simulink model "Spektren_Digitale_Modulation"  (Simulink 8.6)
settings: Solver=FixedStepDiscrete  StartTime=0  StopTime=inf  RelTol=1e-3
undefined symbols (not defined in the file or in its folder): gcbh, magnitude, rcfiltgaincompat
libraries: commfilt2 x6, commrandsrc2 x6, commdigbbndam3 x4, dspstat3 x3, commdigbbndpm3 x2, dspsigops x1, simulink x1
settings Model: Creator=schwall  LastModifiedBy=wunsch
settings DataIOCC: SaveOutput=off  SignalLogging=off  SaveTime=off
settings DebuggingCC: FcnCallInpInsideContextMsg=UseLocalSettings

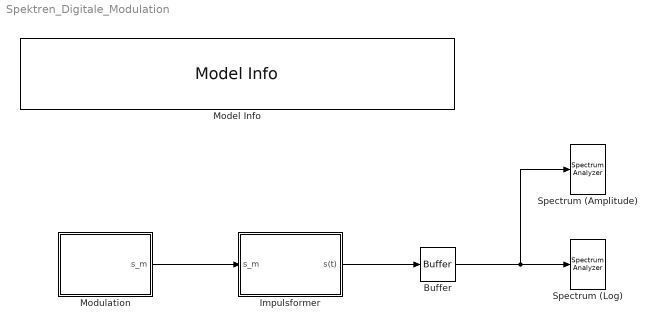
== system Spektren_Digitale_Modulation ==
  Buffer : Buffer  N=1024
  Impulsformer : Subsystem  mask(Impulsformer){rolloff_set=0.4}
      mask prompts: rolloff_set "Root-Raised Cosinus Filter, Roll-Off Faktor:"
      mask help: Impulsformer auswaehlen. Zweiter Vektor ist Rechteckimpulsform.
      mask TypeOptions rolloff_set: 0 | 0.2 | 0.4 | 0.6 | 0.8 | 1
  Model Info : simulink/Model-Wide Utilities/Model Info  BlockCM=None  Frame=on  DisplayStringWithTags=|  HorizontalTextAlignment=Left  LeftAlignmentValue=0.02  SourceBlockDiagram=Spektren_Digitale_Modulation  TagMaxNumber=20
      | Demo Spektren Digitale Modulation
      | Vorlesung Nachrichtentechnik II
      | Institut fuer Nachrichtentechnik (CEL)
  Modulation : Subsystem  mask(Modulation){mod_set=QPSK, mod_prob=0.5, fs=1/100, P=1}
      mask prompts: mod_set "Modulationsverfahren:"; mod_prob "Wahrscheinlichkeit fuer binaere Null:"; fs "Symboldauer [s]:"; P "Leistung, bezogen auf 1 Ohm [Watt]"
      mask help: Modulationsverfahren auswaehlen.
      mask TypeOptions mod_set: 2-ASK | QPSK | 16-PSK | 4-QAM | 16-QAM | 256-QAM
  Spectrum (Amplitude) : SpectrumAnalyzer
  Spectrum (Log) : SpectrumAnalyzer
  wires:
  Modulation/1(s_m) -> Impulsformer/1(s_m)
  Buffer/1 -> Spectrum (Log)/1, Spectrum (Amplitude)/1
  Impulsformer/1(s(t)) -> Buffer/1

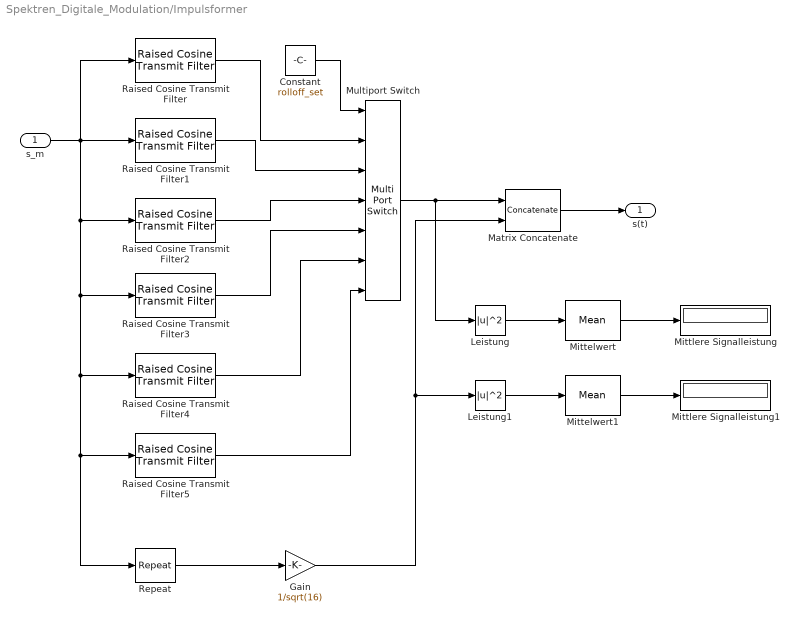
== system Spektren_Digitale_Modulation/Impulsformer ==
  s_m : Inport
  Constant : Constant  Value=rolloff_set
  Gain : Gain  Gain=1/sqrt(16)
  Leistung : Math  Operator=magnitude^2  SaturateOnIntegerOverflow=on
  Leistung1 : Math  Operator=magnitude^2  SaturateOnIntegerOverflow=on
  Matrix Concatenate : Concatenate  Mode=Multidimensional array  ConcatenateDimension=2
  Mittelwert : dspstat3/Mean  run=on  reset_popup=None  InputProcessing=Inherited (this choice will be removed - see release notes)  directionMode=Each column  dimension=1  roiEnable=off  roiType=Rectangles  roiPortion=Entire ROI  roiOutput=Individual statistics for each ROI  roiFlag=off  outputDataTypeStr=Inherit: Same as accumulator  outputLastDataTypeStr=Inherit: Same as accumulator  outputMin=[]  outputMax=[]  roundingMode=Floor  overflowMode=off
  Mittelwert1 : dspstat3/Mean  run=on  reset_popup=None  InputProcessing=Inherited (this choice will be removed - see release notes)  directionMode=Each column  dimension=1  roiEnable=off  roiType=Rectangles  roiPortion=Entire ROI  roiOutput=Individual statistics for each ROI  roiFlag=off  outputDataTypeStr=Inherit: Same as accumulator  outputLastDataTypeStr=Inherit: Same as accumulator  outputMin=[]  outputMax=[]  roundingMode=Floor  overflowMode=off
  Mittlere Signalleistung : Display
  Mittlere Signalleistung1 : Display
  Multiport Switch : MultiPortSwitch  Inputs=6
  Raised Cosine Transmit Filter : commfilt2/Raised Cosine Transmit Filter  filtType=Square root  filtSpan=2*(6)  currentFiltSpan=2*(6)  D=6  R=0  sampMode=Mute  saveAsFlag=0  N=16  framing=Maintain input frame rate  InputProcessing=Columns as channels (frame based)  checkGain=Normalized  filterGain=rcfiltgaincompat(gcbh)  checkCoeff=off  variableName=rcTxFilt  launchFVT=off  roundingMode=Floor  overflowMode=off
  Raised Cosine Transmit Filter1 : commfilt2/Raised Cosine Transmit Filter  filtType=Square root  filtSpan=2*(6)  currentFiltSpan=2*(6)  D=6  R=0.2  sampMode=Mute  saveAsFlag=0  N=16  framing=Maintain input frame rate  InputProcessing=Columns as channels (frame based)  checkGain=Normalized  filterGain=rcfiltgaincompat(gcbh)  checkCoeff=off  variableName=rcTxFilt1  launchFVT=off  roundingMode=Floor  overflowMode=off
  Raised Cosine Transmit Filter2 : commfilt2/Raised Cosine Transmit Filter  filtType=Square root  filtSpan=2*(6)  currentFiltSpan=2*(6)  D=6  R=0.4  sampMode=Mute  saveAsFlag=0  N=16  framing=Maintain input frame rate  InputProcessing=Columns as channels (frame based)  checkGain=Normalized  filterGain=rcfiltgaincompat(gcbh)  checkCoeff=off  variableName=rcTxFilt2  launchFVT=off  roundingMode=Floor  overflowMode=off
  Raised Cosine Transmit Filter3 : commfilt2/Raised Cosine Transmit Filter  filtType=Square root  filtSpan=2*(6)  currentFiltSpan=2*(6)  D=6  R=0.6  sampMode=Mute  saveAsFlag=0  N=16  framing=Maintain input frame rate  InputProcessing=Columns as channels (frame based)  checkGain=Normalized  filterGain=rcfiltgaincompat(gcbh)  checkCoeff=off  variableName=rcTxFilt3  launchFVT=off  roundingMode=Floor  overflowMode=off
  Raised Cosine Transmit Filter4 : commfilt2/Raised Cosine Transmit Filter  filtType=Square root  filtSpan=2*(6)  currentFiltSpan=2*(6)  D=6  R=0.8  sampMode=Mute  saveAsFlag=0  N=16  framing=Maintain input frame rate  InputProcessing=Columns as channels (frame based)  checkGain=Normalized  filterGain=rcfiltgaincompat(gcbh)  checkCoeff=off  variableName=rcTxFilt4  launchFVT=off  roundingMode=Floor  overflowMode=off
  Raised Cosine Transmit Filter5 : commfilt2/Raised Cosine Transmit Filter  filtType=Square root  filtSpan=2*(6)  currentFiltSpan=2*(6)  D=6  R=1  sampMode=Mute  saveAsFlag=0  N=16  framing=Maintain input frame rate  InputProcessing=Columns as channels (frame based)  checkGain=Normalized  filterGain=rcfiltgaincompat(gcbh)  checkCoeff=off  variableName=rcTxFilt5  launchFVT=off  roundingMode=Floor  overflowMode=off
  Repeat : dspsigops/Repeat  N=16  InputProcessing=Inherited (this choice will be removed - see release notes)  RateOptions=Enforce single-rate processing  ic=0  mode=Unused parameter value
  s(t) : Outport
  wires:
  s_m/1 -> Raised Cosine Transmit Filter/1, Raised Cosine Transmit Filter5/1, Repeat/1, Raised Cosine Transmit Filter4/1, Raised Cosine Transmit Filter3/1, Raised Cosine Transmit Filter2/1, Raised Cosine Transmit Filter1/1
  Mittelwert/1 -> Mittlere Signalleistung/1
  Leistung/1 -> Mittelwert/1
  Mittelwert1/1 -> Mittlere Signalleistung1/1
  Leistung1/1 -> Mittelwert1/1
  Multiport Switch/1 -> Matrix Concatenate/1, Leistung/1
  Constant/1 -> Multiport Switch/1
  Raised Cosine Transmit Filter/1 -> Multiport Switch/2
  Raised Cosine Transmit Filter1/1 -> Multiport Switch/3
  Raised Cosine Transmit Filter2/1 -> Multiport Switch/4
  Raised Cosine Transmit Filter3/1 -> Multiport Switch/5
  Raised Cosine Transmit Filter4/1 -> Multiport Switch/6
  Raised Cosine Transmit Filter5/1 -> Multiport Switch/7
  Gain/1 -> Leistung1/1, Matrix Concatenate/2
  Repeat/1 -> Gain/1
  Matrix Concatenate/1 -> s(t)/1

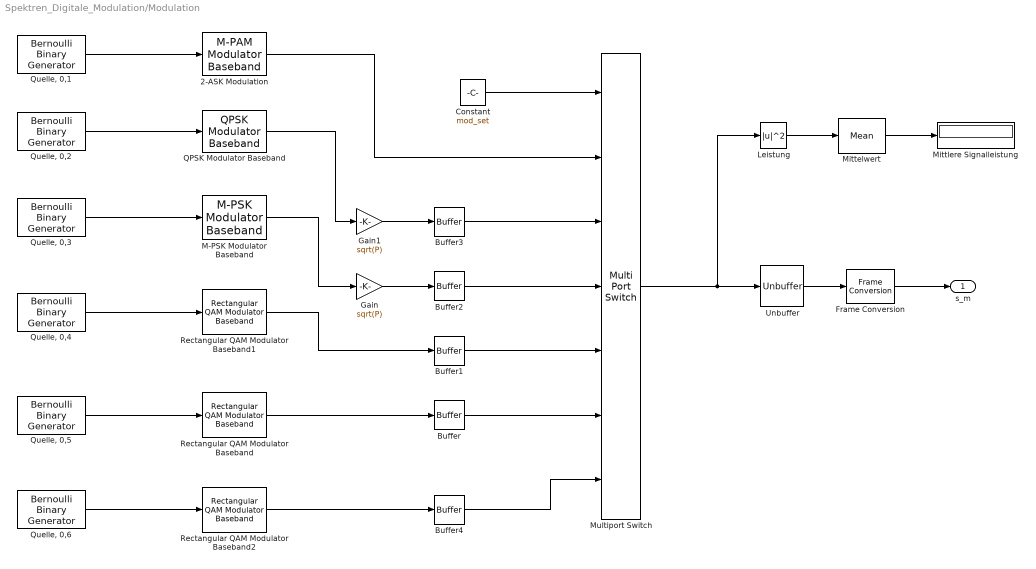
== system Spektren_Digitale_Modulation/Modulation ==
  2-ASK Modulation : commdigbbndam3/M-PAM Modulator Baseband  M=2  InType=Integer  Enc=Binary  PowType=Average Power  MinDist=2  AvgPow=P  PeakPow=1  outDtype=double  outWordLen=16  outUDDataType=sfix(16)  outFracLenMode=Best precision  outFracLen=15
  Buffer{,1..4} (5 alike) : Buffer  N=8
  Constant : Constant  Value=mod_set
  Frame Conversion : FrameConversion  InheritSamplingMode=off
  Gain : Gain  Gain=sqrt(P)
  Gain1 : Gain  Gain=sqrt(P)
  Leistung : Math  Operator=magnitude^2  SaturateOnIntegerOverflow=on
  M-PSK Modulator Baseband : commdigbbndpm3/M-PSK Modulator Baseband  M=16  InType=Bit  Enc=Gray  Mapping=[0:7]  Ph=pi/8  outDtype=double  outWordLen=16  outUDDataType=sfix(16)  outFracLenMode=Best precision  outFracLen=15
  Mittelwert : dspstat3/Mean  run=on  reset_popup=None  InputProcessing=Inherited (this choice will be removed - see release notes)  directionMode=Each column  dimension=1  roiEnable=off  roiType=Rectangles  roiPortion=Entire ROI  roiOutput=Individual statistics for each ROI  roiFlag=off  outputDataTypeStr=Inherit: Same as accumulator  outputLastDataTypeStr=Inherit: Same as accumulator  outputMin=[]  outputMax=[]  roundingMode=Floor  overflowMode=off
  Mittlere Signalleistung : Display
  Multiport Switch : MultiPortSwitch  Inputs=6
  QPSK Modulator Baseband : commdigbbndpm3/QPSK Modulator Baseband  InType=Bit  Enc=Gray  Ph=0  outDtype=double  outWordLen=16  outUDDataType=sfix(16)  outFracLenMode=Best precision  outFracLen=15
  "Quelle, 0,1" : commrandsrc2/Bernoulli Binary Generator  P=mod_prob  seed=61  Ts=fs  frameBased=on  sampPerFrame=8  orient=off  outDataType=double
  "Quelle, 0,2" : commrandsrc2/Bernoulli Binary Generator  P=mod_prob  seed=61  Ts=fs/2  frameBased=on  sampPerFrame=8  orient=off  outDataType=double
  "Quelle, 0,3" : commrandsrc2/Bernoulli Binary Generator  P=mod_prob  seed=61  Ts=fs/4  frameBased=on  sampPerFrame=8  orient=off  outDataType=double
  "Quelle, 0,4" : commrandsrc2/Bernoulli Binary Generator  P=mod_prob  seed=61  Ts=fs/2  frameBased=on  sampPerFrame=8  orient=off  outDataType=double
  "Quelle, 0,5" : commrandsrc2/Bernoulli Binary Generator  P=mod_prob  seed=61  Ts=fs/4  frameBased=on  sampPerFrame=8  orient=off  outDataType=double
  "Quelle, 0,6" : commrandsrc2/Bernoulli Binary Generator  P=mod_prob  seed=61  Ts=fs/8  frameBased=on  sampPerFrame=8  orient=off  outDataType=double
  Rectangular QAM Modulator Baseband : commdigbbndam3/Rectangular QAM Modulator Baseband  M=16  InType=Bit  Enc=Gray  Mapping=[0:15]  PowType=Average Power  MinDist=2  AvgPow=P  PeakPow=1  Ph=0  outDtype=double  outWordLen=16  outUDDataType=sfix(16)  outFracLenMode=Best precision  outFracLen=15
  Rectangular QAM Modulator Baseband1 : commdigbbndam3/Rectangular QAM Modulator Baseband  M=4  InType=Bit  Enc=Gray  Mapping=[0:15]  PowType=Average Power  MinDist=2  AvgPow=P  PeakPow=1  Ph=0  outDtype=double  outWordLen=16  outUDDataType=sfix(16)  outFracLenMode=Best precision  outFracLen=15
  Rectangular QAM Modulator Baseband2 : commdigbbndam3/Rectangular QAM Modulator Baseband  M=256  InType=Bit  Enc=Gray  Mapping=[0:15]  PowType=Average Power  MinDist=2  AvgPow=P  PeakPow=1  Ph=0  outDtype=double  outWordLen=16  outUDDataType=sfix(16)  outFracLenMode=Best precision  outFracLen=15
  Unbuffer : Unbuffer
  s_m : Outport
  wires:
  2-ASK Modulation/1 -> Multiport Switch/2
  QPSK Modulator Baseband/1 -> Gain1/1
  M-PSK Modulator Baseband/1 -> Gain/1
  Rectangular QAM Modulator Baseband1/1 -> Buffer1/1
  Rectangular QAM Modulator Baseband/1 -> Buffer/1
  Constant/1 -> Multiport Switch/1
  "Quelle, 0,1"/1 -> 2-ASK Modulation/1
  "Quelle, 0,2"/1 -> QPSK Modulator Baseband/1
  "Quelle, 0,3"/1 -> M-PSK Modulator Baseband/1
  "Quelle, 0,4"/1 -> Rectangular QAM Modulator Baseband1/1
  "Quelle, 0,5"/1 -> Rectangular QAM Modulator Baseband/1
  Buffer/1 -> Multiport Switch/6
  Buffer1/1 -> Multiport Switch/5
  Buffer2/1 -> Multiport Switch/4
  Buffer3/1 -> Multiport Switch/3
  Rectangular QAM Modulator Baseband2/1 -> Buffer4/1
  "Quelle, 0,6"/1 -> Rectangular QAM Modulator Baseband2/1
  Buffer4/1 -> Multiport Switch/7
  Unbuffer/1 -> Frame Conversion/1
  Frame Conversion/1 -> s_m/1
  Multiport Switch/1 -> Unbuffer/1, Leistung/1
  Mittelwert/1 -> Mittlere Signalleistung/1
  Leistung/1 -> Mittelwert/1
  Gain/1 -> Buffer2/1
  Gain1/1 -> Buffer3/1
